simulink model "Lab6"  (R2016a)
settings: Solver=VariableStepAuto  StartTime=0.0  StopTime=10.0  RelTol=1e-3
settings Model: Creator=gdlau  LastModifiedBy=gdlau

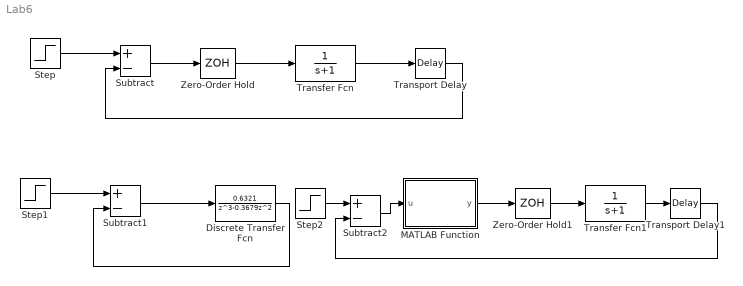
== system Lab6 ==
  Discrete Transfer Fcn : DiscreteTransferFcn  Numerator=[0.6321]  Denominator=[1 -0.3679 0 0]
  MATLAB Function : MATLAB Function  TreatAsAtomicUnit=on
  Step : Step  SampleTime=0
  Step1 : Step  SampleTime=0
  Step2 : Step  SampleTime=0
  Subtract : Sum  Inputs=+-
  Subtract1 : Sum  Inputs=+-
  Subtract2 : Sum  Inputs=+-
  Transfer Fcn : TransferFcn  Denominator=[1 1]
  Transfer Fcn1 : TransferFcn  Denominator=[1 1]
  Transport Delay : TransportDelay
  Transport Delay1 : TransportDelay
  Zero-Order Hold : ZeroOrderHold
  Zero-Order Hold1 : ZeroOrderHold
  wires:
  Step/1 -> Subtract/1
  Subtract/1 -> Zero-Order Hold/1
  Zero-Order Hold/1 -> Transfer Fcn/1
  Transfer Fcn/1 -> Transport Delay/1
  Transport Delay/1 -> Subtract/2
  Subtract1/1 -> Discrete Transfer Fcn/1
  Step1/1 -> Subtract1/1
  Discrete Transfer Fcn/1 -> Subtract1/2
  MATLAB Function/1(y) -> Zero-Order Hold1/1
  Zero-Order Hold1/1 -> Transfer Fcn1/1
  Transfer Fcn1/1 -> Transport Delay1/1
  Transport Delay1/1 -> Subtract2/2
  Step2/1 -> Subtract2/1
  Subtract2/1 -> MATLAB Function/1(u)

== matlab function Lab6/MATLAB Function ==
  data: u input; y output
function y = fcn(u)
%#codegen

y = u;
